simulink model "lecture8_clock"  (Simulink 7.1)
settings: Solver=FixedStepDiscrete  StartTime=0.0  StopTime=20.0  RelTol=1e-3
libraries: simulink x1
settings Model: Creator=pit  LastModifiedBy=pit

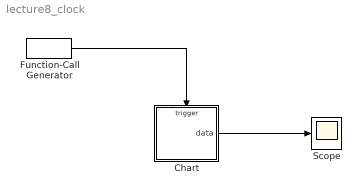
== system lecture8_clock ==
  Chart : Stateflow chart
  Function-Call Generator : simulink/Ports & Subsystems/Function-Call Generator  sample_time=.05  numberOfIterations=1
  Scope : Scope
  wires:
  Function-Call Generator/1 -> Chart/Trigger
  Chart/1(data) -> Scope/1

== stateflow chart Chart ==
  state None
    during: data=data+1
  data: data output double
  events: clock input FUNCTION_CALL_EVENT
